simulink model "RNN_VI"  (R2020b)
settings: Solver=ode3  StartTime=0.0  StopTime=80  FixedStep=5e-4  RelTol=1e-3
settings Model: Creator=ferna  LastModifiedBy=ferna

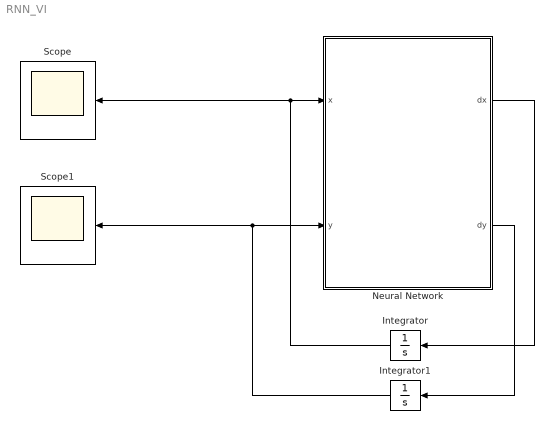
== system RNN_VI ==
  Integrator : Integrator  InitialCondition=[1;-1;2]
  Integrator1 : Integrator  InitialCondition=1
  Neural Network : MATLAB Function  TreatAsAtomicUnit=on
  Scope : Scope
  Scope1 : Scope
  wires:
  Neural Network/1(dx) -> Integrator/1
  Integrator/1 -> Neural Network/1(x), Scope/1
  Neural Network/2(dy) -> Integrator1/1
  Integrator1/1 -> Scope1/1, Neural Network/2(y)

== matlab function RNN_VI/Neural Network ==
  data: x input; dx output; y input; dy output
function [dx,dy] = fcn(x,y)
    
    %%%%%%%%%%%%%%%%%%%%%%%%%%%%%%%%%%%%%%%
    %% Define the Variational Inequality %%
    %%%%%%%%%%%%%%%%%%%%%%%%%%%%%%%%%%%%%%%
    Fx = [5*x(1) + (x(1)+2)^2 + x(2) + x(3) + 10;
          5*x(1) + 3*(x(2)^2) + 10*x(2) + 3*x(3) + 10;
          10*(x(1)+2)^2 + 8*(x(2)^2) + 4*x(3) + 3*(x(3)^2)];       
    %%%%%%%%%%%%%%%%%%%%%%%%
    %% Define Constraints %%
    %%%%%%%%%%%%%%%%%%%%%%%%
    % Inequality Constraints %
    gx = -x(1)-x(2)-x(3)+4;
    dgx1 = -1;          
    dgx2 = -1;
    dgx3 = -1;
    
    dgx = [dgx1;dgx2;dgx3];
       
    %%%%%%%%%%%%%%%%%%%%%%%%%%%%%%
    %% Define Bound Constraints %%
    %%%%%%%%%%%%%%%%%%%%%%%%%%%%%%
    % Upper Bound %
    LowB = [0;0;0]; 
    % Upper bound %
    UpB = [5;5;5]; 

    %%%%%%%%%%%%%%%%%%%%%%%%%%%
    %% Apply the Projections %%
    %%%%%%%%%%%%%%%%%%%%%%%%%%%
    xi = x - Fx - dgx*y;
    
    Px = zeros(length(xi),1);
    for n=1:length(xi)
        Px(n,1) = piecewisex(LowB(n),UpB(n),xi(n)); 
    end
    
    %%%%%%%%%%%%%%%%%%%%%%%%%%%%%%%
    %% Neural Network Structures %%
    %%%%%%%%%%%%%%%%%%%%%%%%%%%%%%%
    dx = -x + Px;
    dy = -y + max(y + gx,0);
end 

%%%%%%%%%%%%%%%%%%%%%%%%%%%%%%%%%%%%
% Evaluation of PieceWise Function %
%%%%%%%%%%%%%%%%%%%%%%%%%%%%%%%%%%%%
% Piecewise Function For States x1, x2, x3 & x4 %
function y = piecewisex(Lbx, Ubx, xin)
    y = 0;
    idx1 = xin <= Lbx;
    y(idx1) = Lbx;
    idx2 = xin >= Ubx;
    y(idx2) = Ubx;
    y(~(idx1 | idx2)) = xin;
end
